simulink model "openloop"  (Simulink 4.00)
settings: Solver=ode45  StartTime=0.0  StopTime=1000  FixedStep=5  RelTol=1e-3
settings Model: LastModifiedBy=bsaunder

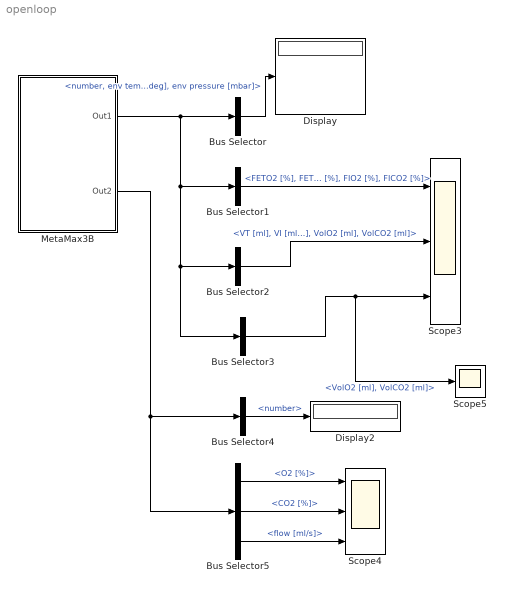
== system openloop ==
  Bus Selector : BusSelector  OutputSignals=number,env temp [deg],env pressure [mbar]  MuxedOutput=on
  Bus Selector1 : BusSelector  OutputSignals=FETO2 [%],FETCO2 [%],FIO2 [%],FICO2 [%]  MuxedOutput=on
  Bus Selector2 : BusSelector  OutputSignals=VT [ml],VI [ml],VolO2 [ml],VolCO2 [ml]  MuxedOutput=on
  Bus Selector3 : BusSelector  OutputSignals=VolO2 [ml],VolCO2 [ml]  MuxedOutput=on
  Bus Selector4 : BusSelector  OutputSignals=number  MuxedOutput=on
  Bus Selector5 : BusSelector  OutputSignals=O2 [%],CO2 [%],flow [ml/s]  MuxedOutput=off
  Display : Display
      settings: Format=short
  Display2 : Display
      settings: Format=short
  MetaMax3B : Subsystem  mask{comport=COM1, Ts=0.1}
      mask prompts: comport "Serial port"; Ts "Sample Time"
      settings: RTWFcnNameOpts=Auto  RTWFileNameOpts=Auto
      mask StyleString: popup(COM1|COM2|COM3|COM4),edit
      mask Display: fprintf('MetaMax 3B\nBreath-by-Breath')
  Scope3 : Scope  NumInputPorts=3
      settings: TimeRange=auto  YMin=0~0~0  YMax=30~3000~600  SaveToWorkspace=off  SaveName=ScopeData  MaxDataPoints=5000
  Scope4 : Scope  NumInputPorts=3
      settings: TimeRange=auto  YMin=17~5.55112e-017~0  YMax=24.5~1.9~900  SaveToWorkspace=off  SaveName=cdat  MaxDataPoints=5000
  Scope5 : Scope
      settings: TimeRange=auto  YMin=-1  YMax=1  SaveToWorkspace=off  SaveName=volO2_volCO2_m_georg  MaxDataPoints=5000
  wires:
  MetaMax3B/1(Out1) -> Bus Selector/1, Bus Selector1/1, Bus Selector2/1, Bus Selector3/1
  Bus Selector/1 -> Display/1  "<number, env temp [deg], env pressure [mbar]>"
  Bus Selector1/1 -> Scope3/1  "<FETO2 [%], FETCO2 [%], FIO2 [%], FICO2 [%]>"
  Bus Selector2/1 -> Scope3/2  "<VT [ml], VI [ml], VolO2 [ml], VolCO2 [ml]>"
  Bus Selector4/1 -> Display2/1  "<number>"
  MetaMax3B/2(Out2) -> Bus Selector4/1, Bus Selector5/1
  Bus Selector5/1 -> Scope4/1  "<O2 [%]>"
  Bus Selector5/2 -> Scope4/2  "<CO2 [%]>"
  Bus Selector5/3 -> Scope4/3  "<flow [ml/s]>"
  Bus Selector3/1 -> Scope3/3, Scope5/1  "<VolO2 [ml], VolCO2 [ml]>"

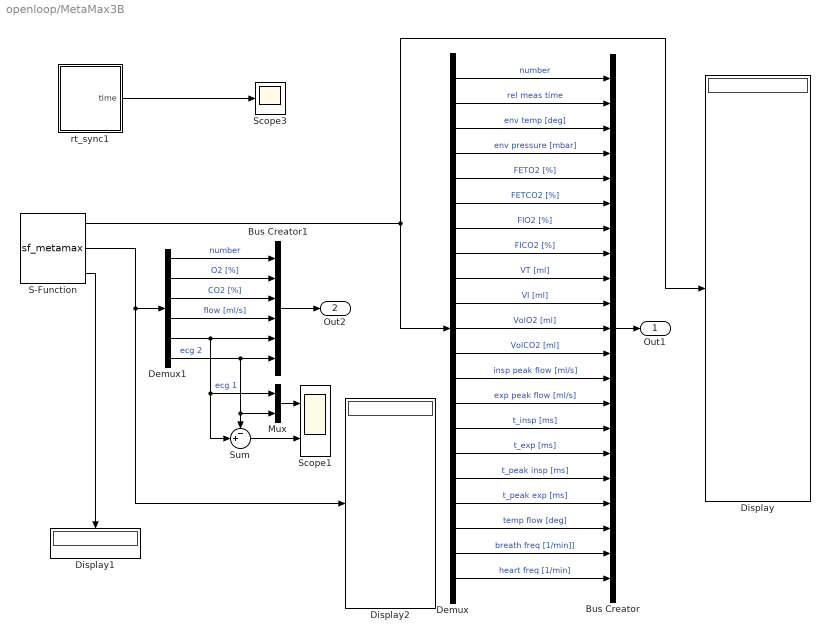
== system openloop/MetaMax3B ==
  Bus Creator : BusCreator  Inputs=21
  Bus Creator1 : BusCreator  Inputs=6
  Demux : Demux  Outputs=21  BusSelectionMode=off
  Demux1 : Demux  Outputs=6  BusSelectionMode=off
  Display : Display
      settings: Format=short
  Display1 : Display
      settings: Orientation=down  Format=short
  Display2 : Display
      settings: Format=short
  Mux : Mux  Inputs=2
  S-Function : S-Function  FunctionName=sf_metamax  Parameters=Ts,comport  PortCounts=[]  SFunctionModules=''
  Scope1 : Scope  NumInputPorts=2
      settings: TimeRange=auto  YMin=7897~-2  YMax=7899~-2  SaveToWorkspace=off  SaveName=hb_m_georg2  MaxDataPoints=5000
  Scope3 : Scope
      settings: TimeRange=auto  YMin=7945  YMax=7962.5  SaveToWorkspace=off  SaveName=hb_m_georg  MaxDataPoints=5000
  Sum : Sum  Inputs=-+|  SaturateOnIntegerOverflow=on
  rt_sync1 : Subsystem  mask{Ts=0.1}
      mask prompts: Ts "Sample Time"
      settings: RTWFcnNameOpts=Auto  RTWFileNameOpts=Auto
      mask Display: fprintf('Real\n Time\n sync')
  Out1 : Outport  Port=1
  Out2 : Outport  Port=2
  wires:
  S-Function/1 -> Demux/1, Display/1
  Demux/1 -> Bus Creator/1  "number"
  Demux/2 -> Bus Creator/2  "rel meas time"
  Demux/3 -> Bus Creator/3  "env temp [deg]"
  Demux/4 -> Bus Creator/4  "env pressure [mbar]"
  Demux/5 -> Bus Creator/5  "FETO2 [%]"
  Demux/6 -> Bus Creator/6  "FETCO2 [%]"
  Demux/7 -> Bus Creator/7  "FIO2 [%]"
  Demux/8 -> Bus Creator/8  "FICO2 [%]"
  Demux/9 -> Bus Creator/9  "VT [ml]"
  Demux/10 -> Bus Creator/10  "VI [ml]"
  Demux/11 -> Bus Creator/11  "VolO2 [ml]"
  Demux/12 -> Bus Creator/12  "VolCO2 [ml]"
  Demux/13 -> Bus Creator/13  "insp peak flow [ml/s]"
  Demux/14 -> Bus Creator/14  "exp peak flow [ml/s]"
  Demux/15 -> Bus Creator/15  "t_insp [ms]"
  Demux/16 -> Bus Creator/16  "t_exp [ms]"
  Demux/17 -> Bus Creator/17  "t_peak insp [ms]"
  Demux/18 -> Bus Creator/18  "t_peak exp [ms]"
  Demux/19 -> Bus Creator/19  "temp flow [deg]"
  Demux/20 -> Bus Creator/20  "breath freq [1/min]]"
  Demux/21 -> Bus Creator/21  "heart freq [1/min]"
  Bus Creator/1 -> Out1/1
  S-Function/3 -> Display1/1
  Demux1/1 -> Bus Creator1/1  "number"
  Demux1/2 -> Bus Creator1/2  "O2 [%]"
  Demux1/3 -> Bus Creator1/3  "CO2 [%]"
  Demux1/4 -> Bus Creator1/4  "flow [ml/s]"
  S-Function/2 -> Demux1/1, Display2/1
  Demux1/5 -> Bus Creator1/5, Mux/1, Sum/2  "ecg 1"
  Demux1/6 -> Bus Creator1/6, Mux/2, Sum/1  "ecg 2"
  Bus Creator1/1 -> Out2/1
  rt_sync1/1(time) -> Scope3/1
  Mux/1 -> Scope1/1
  Sum/1 -> Scope1/2

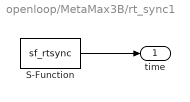
== system openloop/MetaMax3B/rt_sync1 ==
  S-Function : S-Function  FunctionName=sf_rtsync  Parameters=Ts  PortCounts=[]  SFunctionModules=''
  time : Outport  Port=1
  wires:
  S-Function/1 -> time/1
